simulink model "Simulations_section43"  (R2023a)
settings: Solver=ode15s  StartTime=0.0  StopTime=1200  RelTol=1e-3  EnableMultiTasking=on
values from neighbouring files (symbols this model uses):
  bi_j = []    [Section43.m]    (also in ThreeTanks_LPVobserver.m)
  C = [0 0 1]    [Section43.m]    (also in ThreeTanks_LPVobserver.m)
  Q0 = C3*H30^(Alfa3)    (= 0.000130011411968)    [Section43.m]    (also in ThreeTanks_LPVobserver.m)
  vertices = [0.05,0.7;0.03,1.5;0.03,1.1;0.03,1.4;0.03,1.8]    [Section43.m]    (also in ThreeTanks_LPVobserver.m)
  x0 = [H10;H20;H30]    [Section43.m]    (also in ThreeTanks_LPVobserver.m)
  xest0 = 0.5*x0    [Section43.m]    (also in ThreeTanks_LPVobserver.m)
undefined symbols (not defined in the file or in its folder): Aobs, Bobs
settings Model: Creator=a217456  LastModifiedBy=senameo
settings SolverCC: AlgebraicLoopSolver=TrustRegion
settings DataIOCC: LimitDataPoints=on  ReturnWorkspaceOutputs=off
settings OptimizationCC: LifeSpan=inf
settings DebuggingCC: UnconnectedInputMsg=warning  UnconnectedOutputMsg=warning  UnconnectedLineMsg=warning  AllowSymbolicDim=off  SFUnexpectedBacktrackingDiag=warning  SFNoUnconditionalDefaultTransitionDiag=warning  SFExecutionAtInitializationDiag=none  ArithmeticOperatorsInVariantConditions=warning
settings ModelReferenceCC: EnableRefExpFcnMdlSchedulingChecks=on  PropagateSignalLabelsOutOfModel=off
settings SFSimCC: SimUseLocalCustomCode=off  CustomCodeUndefinedFunction=UseInterfaceOnly
settings RTWCC: RTWUseLocalCustomCode=off  DLArmComputeVersion=19.05
settings CodeAppCC: StateflowObjectComments=on
settings GRTTargetCC: TargetLangStandard=C89/C90 (ANSI)
settings ConfigComp: CovMetricSettings=dw  CovSaveCumulativeToWorkspaceVar=on  CovSaveSingleToWorkspaceVar=on  CovExternalEMLEnable=off

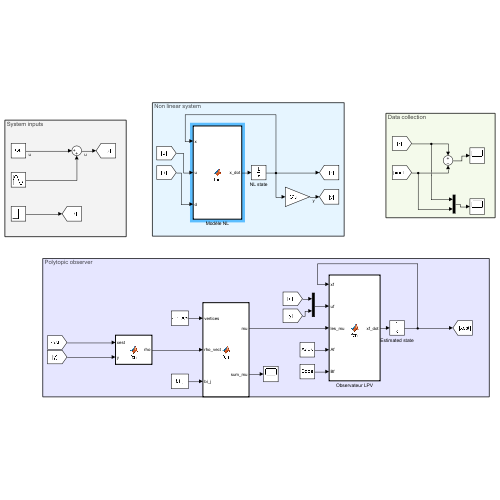
[thumbnail: Simulink's stored preview of the top-level diagram]
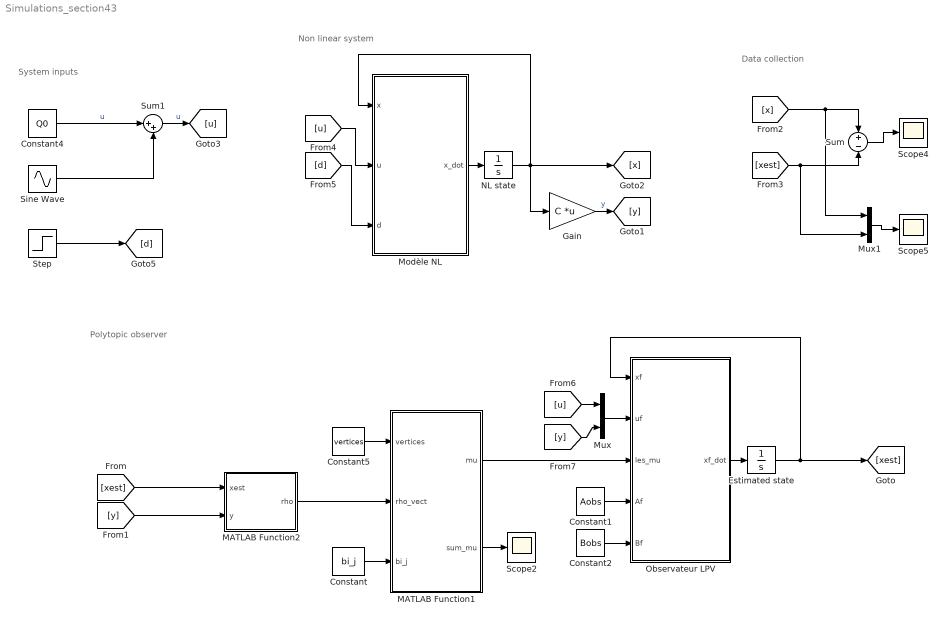
== system Simulations_section43 ==
  note: Data collection
  note: Non linear system
  note: System inputs
  note: Polytopic observer
  Constant : Constant  Value=bi_j
  Constant1 : Constant  Value=Aobs
  Constant2 : Constant  Value=Bobs
  Constant4 : Constant  Value=Q0
  Constant5 : Constant  Value=vertices  VectorParams1D=off
  Estimated state : Integrator  InitialCondition=xest0
  Gain : Gain  Gain=C  Multiplication=Matrix(K*u)
  MATLAB Function1 : MATLAB Function  TreatAsAtomicUnit=on
  MATLAB Function2 : MATLAB Function  TreatAsAtomicUnit=on
  Modèle NL : MATLAB Function  TreatAsAtomicUnit=on
  Mux : Mux  Inputs=2
  Mux1 : Mux  Inputs=2
  NL state : Integrator  InitialCondition=x0
  Observateur LPV : MATLAB Function  TreatAsAtomicUnit=on
  Scope2 : Scope
  Scope4 : Scope
  Scope5 : Scope
  Sine Wave : Sin  Amplitude=-1e-5  Frequency=0.005  SampleTime=0
  Step : Step  Time=600  After=1e-5  SampleTime=0
  Sum : Sum  Inputs=+-
  Sum1 : Sum  Inputs=|++
  wires:
  Constant/1 -> MATLAB Function1/3(bi_j)
  MATLAB Function1/1(mu) -> Observateur LPV/3(les_mu)
  Observateur LPV/1(xf_dot) -> Estimated state/1
  Constant1/1 -> Observateur LPV/4(Af)
  Constant2/1 -> Observateur LPV/5(Bf)
  Constant5/1 -> MATLAB Function1/1(vertices)
  Mux/1 -> Observateur LPV/2(uf)
  Gain/1 -> [y]  "y"
  Modèle NL/1(x_dot) -> NL state/1
  NL state/1 -> Gain/1, [x], Modèle NL/1(x)
  MATLAB Function1/2(sum_mu) -> Scope2/1
  Constant4/1 -> Sum1/1  "u"
  Sine Wave/1 -> Sum1/2
  Estimated state/1 -> Observateur LPV/1(xf), [xest]
  [xest] -> MATLAB Function2/1(xest)
  [y] -> MATLAB Function2/2(y)
  MATLAB Function2/1(rho) -> MATLAB Function1/2(rho_vect)
  Sum/1 -> Scope4/1
  Mux1/1 -> Scope5/1
  [x] -> Mux1/1, Sum/1
  [xest] -> Mux1/2, Sum/2
  Sum1/1 -> [u]  "u"
  Step/1 -> [d]
  [u] -> Modèle NL/2(u)
  [d] -> Modèle NL/3(d)
  [u] -> Mux/1
  [y] -> Mux/2

== matlab function Simulations_section43/Observateur LPV ==
  data: xf input; uf input; xf_dot output; les_mu input; Af input; Bf input
function xf_dot  = fcn(xf,uf,les_mu,Af,Bf)

TwopN = length(les_mu);

xf_dot = zeros(size(Af(:,:,1),1),1);

for i=1:TwopN
    xf_dot = xf_dot + les_mu(i)*(Af(:,:,i)*xf + Bf(:,:,i)*uf);
end
end

== matlab function Simulations_section43/MATLAB Function1 ==
  data: vertices input; rho_vect input; mu output; bi_j input; sum_mu output
function [mu,sum_mu]  = fcn(vertices,rho_vect,bi_j)
% Algorithm 2 to compute the polytopic coordinates

N = size(vertices,1);

mu = ones(2^N,1);
sum_mu =0;
for i=1:2^N
    for j=1:N
        if bi_j(i,N+1-j) == 0
            alphai_j = 1;
            betai_j = -vertices(j,2);
        else
            alphai_j = -1;
            betai_j = vertices(j,1);
        end
        mu(i) =  mu(i)*((alphai_j*rho_vect(j) + betai_j)/(vertices(j,1)-vertices(j,2)));
    end
    sum_mu = sum_mu+mu(i);
end

end

== matlab function Simulations_section43/Modèle NL ==
  data: x input; u input; d input; x_dot output
function x_dot = fcn(x,u,d)
x1=x(1);
x2=x(2);
x3=x(3);
a=25*10^(-2);
b=34.5*10^(-2);
c=10*10^(-2);
w=3.5*10^(-2);
R=36.4*10^(-2);
L=35*10^(-2);
%tank section
S1=a*w;
S2=w*(c+x2/L*b);
S3=w*sqrt(R^2-(R-x3)^2);
% model parameters
C1=2.3314e-04; 
C2=2.7312e-04;
C3=2.4837e-04;
Alfa1=0.3068; 
Alfa2=0.4120; 
Alfa3=0.3412;

%
x_dot1=(u-C1*x1^(Alfa1)+0.1*d)/S1;
x_dot2=(C1*x1^(Alfa1)-C2*x2^(Alfa2))/S2;
x_dot3=(C2*x2^(Alfa2)-C3*x3^(Alfa3))/S3;
x_dot = [x_dot1;x_dot2;x_dot3];

end

== matlab function Simulations_section43/MATLAB Function2 ==
  data: xest input; rho output; y input
function rho = fcn(xest,y)
x1hat=xest(1);
x2hat=xest(2);
x3hat=xest(3);
% parameters
a=25*10^(-2);
b=34.5*10^(-2);
c=10*10^(-2);
w=3.5*10^(-2);
R=36.4*10^(-2);
L=35*10^(-2);
C1=2.3314e-04; 
C2=2.7312e-04;
C3=2.4837e-04;
Alfa1=0.3068; 
Alfa2=0.4120; 
Alfa3=0.3412;
S1=a*w;
S2=w*(c+x2hat/L*b);
S3=w*sqrt(R^2-(R-y)^2);
% estimated scheduling parameters
rho1=C1/S1*x1hat^(Alfa1-1);
rho2=C1/S2*x1hat^(Alfa1-1);
rho3=C2/S2*x2hat^(Alfa2-1);
rho4=C2/S3*x2hat^(Alfa2-1);
rho5=C3/S3*y^(Alfa3-1);  % x3 is measured y=x3
rho=[rho1;rho2;rho3;rho4;rho5];
